simulink model "assignment1"  (R2024a)
settings: Solver=VariableStepAuto  StartTime=0.0  StopTime=10.0  RelTol=1e-3
settings Model: Creator=robin  LastModifiedBy=robin

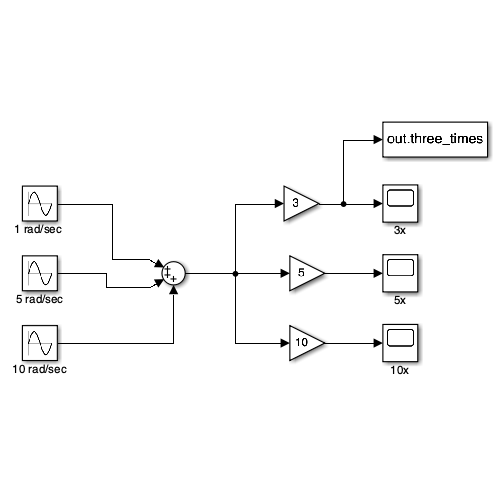
[thumbnail: Simulink's stored preview of the top-level diagram]
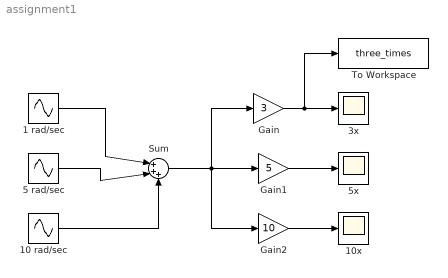
== system assignment1 ==
  "1 rad/sec " : Sin  SampleTime=0
  10 rad/sec : Sin  SampleTime=0
  10x : Scope
  3x : Scope
  5 rad/sec : Sin  SampleTime=0
  5x : Scope
  Gain : Gain  Gain=3
  Gain1 : Gain  Gain=5
  Gain2 : Gain  Gain=10
  Sum : Sum  Inputs=|+++
  To Workspace : ToWorkspace  VariableName=three_times  SaveFormat=Timeseries  SampleTime=-1
  wires:
  "1 rad/sec "/1 -> Sum/1
  5 rad/sec/1 -> Sum/2
  10 rad/sec/1 -> Sum/3
  Sum/1 -> Gain2/1, Gain1/1, Gain/1
  Gain/1 -> To Workspace/1, 3x/1
  Gain1/1 -> 5x/1
  Gain2/1 -> 10x/1
